simulink model "sweep_testbench"  (Simulink 8.9)
settings: Solver=ode45  StartTime=0.0  StopTime=simu.trantime  FixedStep=1/Fs  RelTol=1e-3  EnableMultiTasking=on
undefined symbols (not defined in the file): dc, Fs, OSR, simu, sinamp, sinfreq
libraries: dsparch4 x1, dspsrcs4 x1, simulink x1
settings Model: Creator=amyles  LastModifiedBy=Arnaldi Isacco
settings SolverCC: AutoInsertRateTranBlk=on
settings DataIOCC: LimitDataPoints=off  SaveOutput=off  SignalLogging=off  DSMLogging=off  SaveTime=off
settings OptimizationCC: ExpressionDepthLimit=2147483647
settings DebuggingCC: StrictBusMsg=Warning
settings ModelReferenceCC: ModelReferenceNumInstancesAllowed=Single

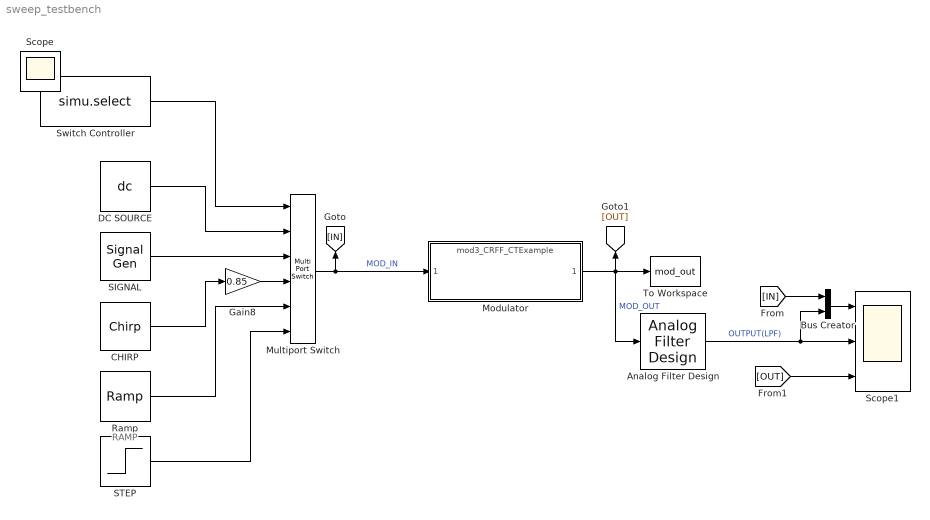
== system sweep_testbench ==
  note: RAMP
  Analog Filter Design : dsparch4/Analog Filter Design  method=Butterworth  filttype=Lowpass  N=8  Wlo=pi*(Fs/OSR)  Whi=80  Rp=2  Rs=40
      settings: AttributesFormatString=Low-pass filter the loop output\nto illustrate intuitively how the\npulse density modulated +1/-1\noutput stream does capture\nthe input signal
  Bus Creator : BusCreator  Inputs=2
  CHIRP : dspsrcs4/Chirp  sweep=Linear  mode=Unidirectional  f0=1  f1=Fs/(OSR)  t1=simu.trantime/10  Tsweep=simu.trantime/10  phase=0  Ts=1/Fs  spf=1  datatype=Double  OutputFrames=on
      settings: SourceProductName=DSP System Toolbox
  DC SOURCE : Constant  Value=dc  SampleTime=1/Fs
  Gain8 : Gain  Gain=0.85  SampleTime=1/Fs
  Modulator : ModelReference  ModelNameDialog=mod3_CRFF_CTExample.mdl  SimulationMode=Normal  ModelReferenceVersion=1.122
  Multiport Switch : MultiPortSwitch  Inputs=5  SampleTime=1/Fs
  Ramp : simulink/Sources/Ramp  slope=140  start=1/300  X0=0
  SIGNAL : SignalGenerator  Amplitude=sinamp  Frequency=sinfreq  VectorParams1D=off
  STEP : Step  Time=9.6e-3  After=0.88  SampleTime=0
  Scope1 : Scope  NumInputPorts=3
  Switch Controller : Constant  Value=simu.select  SampleTime=1/Fs
  To Workspace : ToWorkspace  VariableName=mod_out  SampleTime=1/Fs
      settings: MaxDataPoints=50000000
  Scope : Scope
  wires:
  Modulator/1 -> To Workspace/1, Analog Filter Design/1, [OUT]  "MOD_OUT"
  Multiport Switch/1 -> Modulator/1, [IN]  "MOD_IN"
  Switch Controller/1 -> Multiport Switch/1
  DC SOURCE/1 -> Multiport Switch/2
  SIGNAL/1 -> Multiport Switch/3
  Ramp/1 -> Multiport Switch/5
  [OUT] -> Scope1/3
  Analog Filter Design/1 -> Scope1/2, Bus Creator/2  "OUTPUT(LPF)"
  Gain8/1 -> Multiport Switch/4
  CHIRP/1 -> Gain8/1
  STEP/1 -> Multiport Switch/6
  Bus Creator/1 -> Scope1/1
  [IN] -> Bus Creator/1
